simulink model "untitled2"  (Simulink 7.4)
settings: Solver=ode45  StartTime=0.0  StopTime=10.0  RelTol=1e-3
libraries: dspinverses x1, dspsolvers x1
settings Model: Creator=autologin  LastModifiedBy=autologin

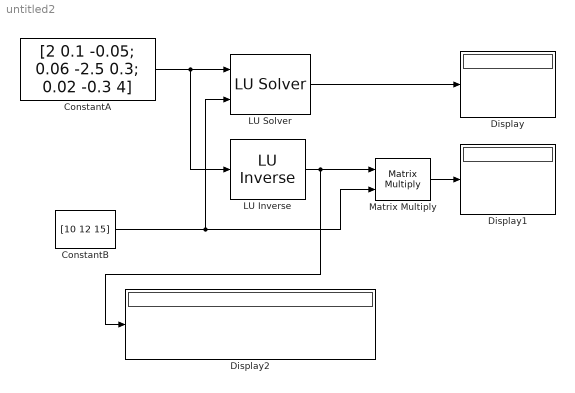
== system untitled2 ==
  " LU Inverse" : dspinverses/ LU Inverse  SystemSampleTime=-1
  ConstantA : Constant  Value=[2 0.1 -0.05; 0.06 -2.5 0.3; 0.02 -0.3 4]  OutDataType=fixdt(1, 16)  OutScaling=2^0
  ConstantB : Constant  Value=[10 12 15]  OutDataType=fixdt(1, 16)  OutScaling=2^0
  Display : Display
  Display1 : Display
  Display2 : Display
  LU Solver : dspsolvers/LU Solver  SystemSampleTime=-1
  Matrix Multiply : Product  Multiplication=Matrix(*)  OutDataType=sfix(16)  OutScaling=2^0
  wires:
  ConstantA/1 -> LU Solver/1, " LU Inverse"/1
  ConstantB/1 -> Matrix Multiply/2, LU Solver/2
  " LU Inverse"/1 -> Matrix Multiply/1, Display2/1
  LU Solver/1 -> Display/1
  Matrix Multiply/1 -> Display1/1
